simulink model "Suspension_sys"  (R2020b)
settings: Solver=VariableStepAuto  StartTime=0.0  StopTime=10  RelTol=1e-3
values from neighbouring files (symbols this model uses):
  b1 = 350    [parameters.m]
  b2 = 15020    [parameters.m]
  k1 = 80000    [parameters.m]
  k2 = 500000    [parameters.m]
  m1 = 2500    [parameters.m]
  m2 = 320    [parameters.m]
settings Model: Creator=Abhinav dixit  LastModifiedBy=Abhinav dixit

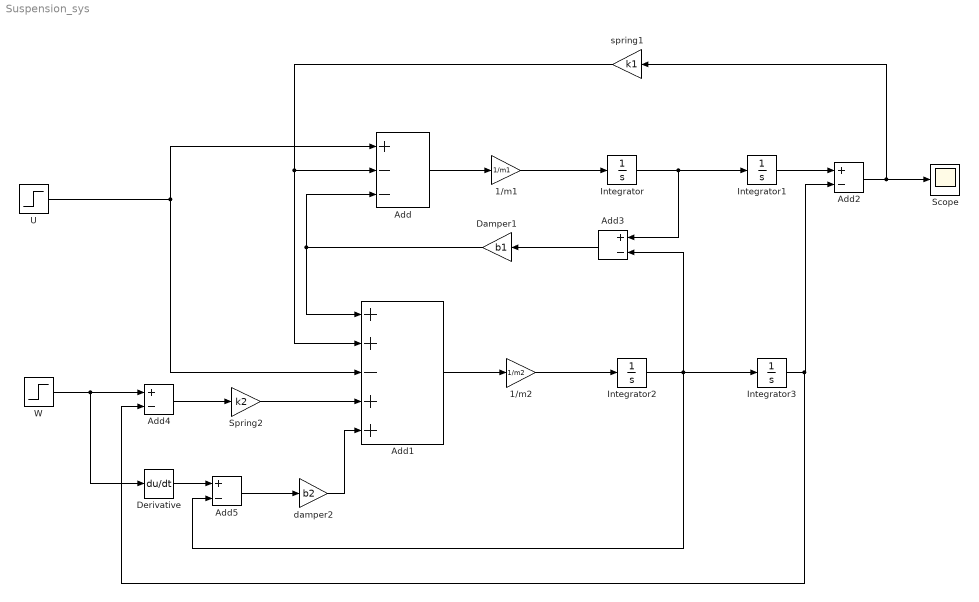
== system Suspension_sys ==
  1/m1 : Gain  Gain=1/m1
  1/m2 : Gain  Gain=1/m2
  Add : Sum  Inputs=+--
  Add1 : Sum  Inputs=++-++
  Add{2..5} (4 alike) : Sum  Inputs=+-
  Damper1 : Gain  Gain=b1
  Derivative : Derivative
  Integrator{,1..3} (4 alike) : Integrator
  Scope : Scope
  Spring2 : Gain  Gain=k2
  U : Step  SampleTime=0
  W : Step  Time=0  After=0  SampleTime=0
  damper2 : Gain  Gain=b2
  spring1 : Gain  Gain=k1
  wires:
  1/m1/1 -> Integrator/1
  Integrator/1 -> Add3/1, Integrator1/1
  Integrator2/1 -> Add5/2, Add3/2, Integrator3/1
  1/m2/1 -> Integrator2/1
  Add1/1 -> 1/m2/1
  Add/1 -> 1/m1/1
  Integrator1/1 -> Add2/1
  spring1/1 -> Add/2, Add1/2
  Add2/1 -> Scope/1, spring1/1
  Integrator3/1 -> Add4/2, Add2/2
  Damper1/1 -> Add1/1, Add/3
  Add3/1 -> Damper1/1
  Spring2/1 -> Add1/4
  Add4/1 -> Spring2/1
  W/1 -> Derivative/1, Add4/1
  Add5/1 -> damper2/1
  Derivative/1 -> Add5/1
  damper2/1 -> Add1/5
  U/1 -> Add/1, Add1/3
